simulink model "InjCrv_PoI2AddCor"  (R2016b)
settings: configuration reference "CodeGenConfigSet" (kept outside this file)
values from neighbouring files (symbols this model uses):
  ETCtl_qPoI2_C = Calibration.Parameter    [init_InjCrv_PoI2AddCor.m]
  InjCrv_phiAddCorRmt_C = Calibration.Parameter    [init_InjCrv_PoI2AddCor.m]
  InjCrv_phiPoI2_C = Calibration.Parameter    [init_InjCrv_PoI2AddCor.m]
  InjCrv_qPoI2_C = Calibration.Parameter    [init_InjCrv_PoI2AddCor.m]
  InjCrv_qPoI2Eff_C = Calibration.Parameter    [init_InjCrv_PoI2AddCor.m]
  InjCrv_stInjCharSetVal_C = Calibration.Parameter    [init_InjCrv_PoI2AddCor.m]
  InjCrv_swtPhiAddCorRmt_C = Calibration.Parameter    [init_InjCrv_PoI2AddCor.m]
  InjCrv_swtPoI2ETCtl_C = Calibration.Parameter    [init_InjCrv_PoI2AddCor.m]
  InjCrv_swtPoI2FMTC_C = Calibration.Parameter    [init_InjCrv_PoI2AddCor.m]
  InjCrv_swtPoI2Phi_C = Calibration.Parameter    [init_InjCrv_PoI2AddCor.m]
  InjCrv_swtPoI2Q_C = Calibration.Parameter    [init_InjCrv_PoI2AddCor.m]
  InjCrv_swtPoI2QEff_C = Calibration.Parameter    [init_InjCrv_PoI2AddCor.m]
  InjCrv_swtPoI2Ti_C = Calibration.Parameter    [init_InjCrv_PoI2AddCor.m]
  InjCrv_swtTiAddCorRmt_C = Calibration.Parameter    [init_InjCrv_PoI2AddCor.m]
  InjCrv_tiAddCorRmt_C = Calibration.Parameter    [init_InjCrv_PoI2AddCor.m]
  InjCrv_tiPoI2_C = Calibration.Parameter    [init_InjCrv_PoI2AddCor.m]
undefined symbols (not defined in the file or in its folder): Switch_conv
libraries: simulink x2
settings Model: Creator=Administrator  LastModifiedBy=Wei Liang
settings ConfigSetRef: SourceLocation=Base Workspace

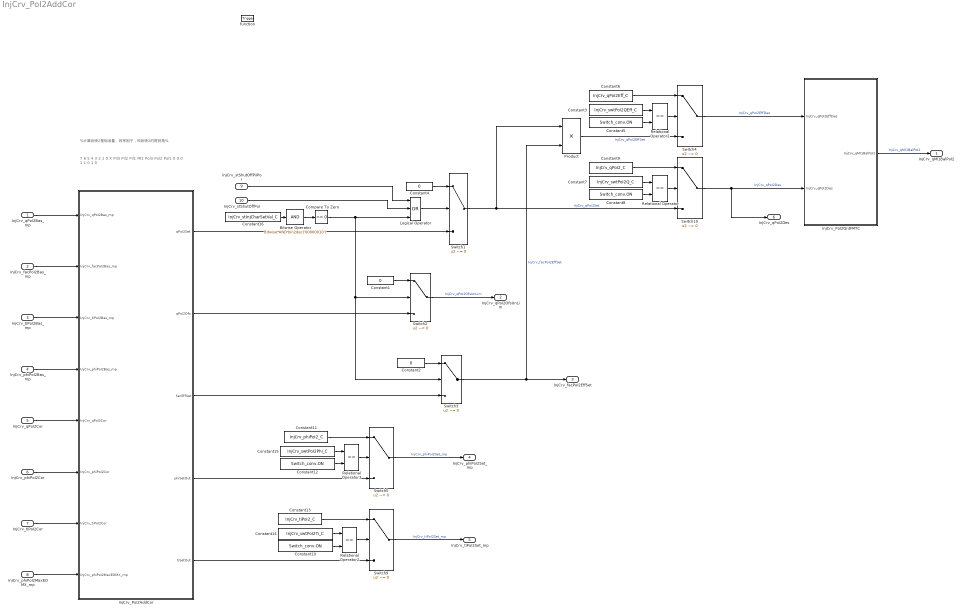
== system InjCrv_PoI2AddCor ==
  note: %计算后喷2基础油量，效率因子，和后喷2的提前角%
  note: 7
      | 6
      | 5
      | 4
      | 3
      | 2
      | 1
      | 0
      |
      | X
      | Pil3
      | Pil2
      | Pil1
      | MI1
      | Pol3
      | Pol2
      | Pol1
      |
      | 0
      | 0
      | 0
      | 1
      | 1
      | 0
      | 1
      | 0
  InjCrv_qPoI2Bas_mp : Inport  Tag=mg/hub  Description=PoI2 base quantity for injection  OutMin=-319  OutMax=319  OutDataTypeStr=FuelMass_mg_hub
  InjCrv_facPoI2Bas_mp : Inport  Description=PoI2 base Efficiency factor  Port=2  OutMin=-10  OutMax=10  OutDataTypeStr=Factor
  InjCrv_tiPoI2Bas_mp : Inport  Tag=us  Description=PoI2 base start of energizing of time  Port=3  OutMin=-13107  OutMax=13106  OutDataTypeStr=InjTime_us
  InjCrv_phiPoI2Bas_mp : Inport  Tag=CA  Description=PoI2 base start of energizing of angle  Port=4  OutMin=-719  OutMax=719  OutDataTypeStr=Angle_CA
  InjCrv_qPoI2Cor : Inport  Tag=mg/hub  Description=PoI2 correction quantity  Port=5  OutMin=-319  OutMax=319  OutDataTypeStr=FuelMass_mg_hub
  InjCrv_phiPoI2Cor : Inport  Tag=CA  Description=PoI2 start of energizing correction angle  Port=6  OutMin=-719  OutMax=719  OutDataTypeStr=Angle_CA
  InjCrv_tiPoI2Cor : Inport  Tag=us  Description=PoI2 start of energizing correction time  Port=7  OutMin=-13107  OutMax=13106  OutDataTypeStr=InjTime_us
  InjCrv_phiPoI2MaxEOMX_mp : Inport  Tag=CA  Description=Maximum PoI2 start of energizing for EOM1-EOM7  Port=8  OutMin=-719  OutMax=719  OutDataTypeStr=Angle_CA
  InjCrv_stShutOffPiIPoI : Inport  Description=State of MI1 fuelMass too small  Port=9  OutMin=0  OutMax=1  OutDataTypeStr=boolean
  InjCrv_stShutOffPoI : Inport  Description=State of MI1 fuelMass too small  Port=10  OutMin=0  OutMax=1  OutDataTypeStr=boolean
  function : TriggerPort  TriggerType=function-call  VariantControl=Variant
  Bitwise Operator : simulink/Logic and Bit Operations/Bitwise Operator  logicop=AND  UseBitMask=on  BitMask=bin2dec('00000010')  BitMaskRealWorld=Stored Integer
  Compare To Zero : simulink/Logic and Bit Operations/Compare To Zero  relop===  OutDataTypeStr=boolean
  Constant1 : Constant  Value=0  OutDataTypeStr=Inherit: Inherit via back propagation
  Constant{5,8,10,12} (4 alike) : Constant  Value=Switch_conv.ON
  Constant11 : Constant  Value=InjCrv_phiPoI2_C
  Constant13 : Constant  Value=InjCrv_tiPoI2_C
  Constant14 : Constant  Value=InjCrv_swtPoI2Ti_C
  Constant15 : Constant  Value=InjCrv_swtPoI2Phi_C
  Constant16 : Constant  Value=InjCrv_stInjCharSetVal_C
  Constant2 : Constant  Value=0  OutDataTypeStr=Inherit: Inherit via back propagation
  Constant3 : Constant  Value=InjCrv_swtPoI2QEff_C
  Constant4 : Constant  Value=0  OutDataTypeStr=Inherit: Inherit via back propagation
  Constant6 : Constant  Value=InjCrv_qPoI2Eff_C
  Constant7 : Constant  Value=InjCrv_swtPoI2Q_C
  Constant9 : Constant  Value=InjCrv_qPoI2_C
  InjCrv_PoI2AddCor : Subsystem  RTWFcnName=InjCrv_PoI2AddCor_Co  RTWFileName=InjCrv_PoI2AddCor
      settings: RTWSystemCode=Nonreusable function  RTWFcnNameOpts=User specified  RTWFileNameOpts=User specified
  InjCrv_PoI2QntFMTC : Subsystem
  Logical Operator : Logic  Operator=OR  Inputs=3  AllPortsSameDT=off  OutDataTypeStr=boolean
  Product : Product  OutDataTypeStr=Inherit: Inherit via back propagation  SaturateOnIntegerOverflow=on
  Relational Operator{,1..3} (4 alike) : RelationalOperator  Operator===  OutDataTypeStr=boolean  RndMeth=Simplest
  Switch{1..5,9..10} (7 alike) : Switch  Criteria=u2 ~= 0
  InjCrv_qMI1BalPoI2 : Outport  Tag=mg/hub  Description=Actual PoI2 quantity contained in FMTC (used for MI1 balance)  OutMin=-319  OutMax=319  OutDataTypeStr=FuelMass_mg_hub
  InjCrv_qPoI2OfsUnLim : Outport  Tag=mg/hub  Description=Unlimited PoI2 offset quantity  Port=2  OutMin=-319  OutMax=319  OutDataTypeStr=FuelMass_mg_hub
  InjCrv_facPoI2EffSet : Outport  Description=Factor for torque forming part of PoI2 injection quantity (setpoint)  Port=3  OutMin=-10  OutMax=10  OutDataTypeStr=Factor
  InjCrv_phiPoI2Set_mp : Outport  Tag=CA  Description=start of energizing Agngle for PoI2  Port=4  OutMin=-719  OutMax=719  OutDataTypeStr=Angle_CA
  InjCrv_tiPoI2Set_mp : Outport  Tag=us  Description=start of energizing time for PoI2  Port=5  OutMin=-13107  OutMax=13106  OutDataTypeStr=InjTime_us
  InjCrv_qPoI2Des : Outport  Tag=mg/hub  Description=Desired PoI2 injection quantity  Port=6  OutMin=-319  OutMax=319  OutDataTypeStr=FuelMass_mg_hub
  wires:
  InjCrv_qPoI2Cor/1 -> InjCrv_PoI2AddCor/5(InjCrv_qPoI2Cor)
  InjCrv_phiPoI2Cor/1 -> InjCrv_PoI2AddCor/6(InjCrv_phiPoI2Cor)
  InjCrv_tiPoI2Cor/1 -> InjCrv_PoI2AddCor/7(InjCrv_tiPoI2Cor)
  InjCrv_PoI2AddCor/1(qPoI2Set) -> Switch1/3
  Switch5/1 -> InjCrv_phiPoI2Set_mp/1  "InjCrv_phiPoI2Set_mp"
  Switch9/1 -> InjCrv_tiPoI2Set_mp/1  "InjCrv_tiPoI2Set_mp"
  Switch1/1 -> Product/1, Switch10/3  "InjCrv_qPoI2Set"
  Bitwise Operator/1 -> Compare To Zero/1
  Constant16/1 -> Bitwise Operator/1
  Constant4/1 -> Switch1/1
  Switch2/1 -> InjCrv_qPoI2OfsUnLim/1  "InjCrv_qPoI2OfsUnLim"
  InjCrv_PoI2AddCor/2(qPoI2Ofs) -> Switch2/3
  InjCrv_PoI2AddCor/3(facEffSet) -> Switch3/3
  Switch3/1 -> InjCrv_facPoI2EffSet/1, Product/2  "InjCrv_facPoI2EffSet"
  Product/1 -> Switch4/3  "InjCrv_qPoI2EffSet"
  Constant6/1 -> Switch4/1
  Constant3/1 -> Relational Operator1/1
  Constant5/1 -> Relational Operator1/2
  Relational Operator1/1 -> Switch4/2
  Switch4/1 -> InjCrv_PoI2QntFMTC/1(InjCrv_qPoI2EffDes)  "InjCrv_qPoI2EffDes"
  Constant9/1 -> Switch10/1
  Constant7/1 -> Relational Operator/1
  Constant8/1 -> Relational Operator/2
  Relational Operator/1 -> Switch10/2
  Switch10/1 -> InjCrv_qPoI2Des/1, InjCrv_PoI2QntFMTC/2(InjCrv_qPoI2Des)  "InjCrv_qPoI2Des"
  Constant10/1 -> Relational Operator2/2
  Relational Operator2/1 -> Switch9/2
  Constant12/1 -> Relational Operator3/2
  Relational Operator3/1 -> Switch5/2
  InjCrv_PoI2AddCor/4(phiSetOut) -> Switch5/3
  InjCrv_PoI2AddCor/5(tiSetOut) -> Switch9/3
  Constant14/1 -> Relational Operator2/1
  Constant13/1 -> Switch9/1
  Constant11/1 -> Switch5/1
  Constant15/1 -> Relational Operator3/1
  Logical Operator/1 -> Switch1/2
  Compare To Zero/1 -> Logical Operator/3, Switch3/2, Switch2/2
  Constant1/1 -> Switch2/1
  Constant2/1 -> Switch3/1
  InjCrv_stShutOffPoI/1 -> Logical Operator/2
  InjCrv_stShutOffPiIPoI/1 -> Logical Operator/1
  InjCrv_PoI2QntFMTC/1(InjCrv_qMI1BalPoI2) -> InjCrv_qMI1BalPoI2/1  "InjCrv_qMI1BalPoI2"
  InjCrv_phiPoI2Bas_mp/1 -> InjCrv_PoI2AddCor/4(InjCrv_phiPoI2Bas_mp)
  InjCrv_tiPoI2Bas_mp/1 -> InjCrv_PoI2AddCor/3(InjCrv_tiPoI2Bas_mp)
  InjCrv_facPoI2Bas_mp/1 -> InjCrv_PoI2AddCor/2(InjCrv_facPoI2Bas_mp)
  InjCrv_qPoI2Bas_mp/1 -> InjCrv_PoI2AddCor/1(InjCrv_qPoI2Bas_mp)
  InjCrv_phiPoI2MaxEOMX_mp/1 -> InjCrv_PoI2AddCor/8(InjCrv_phiPoI2MaxEOMX_mp)

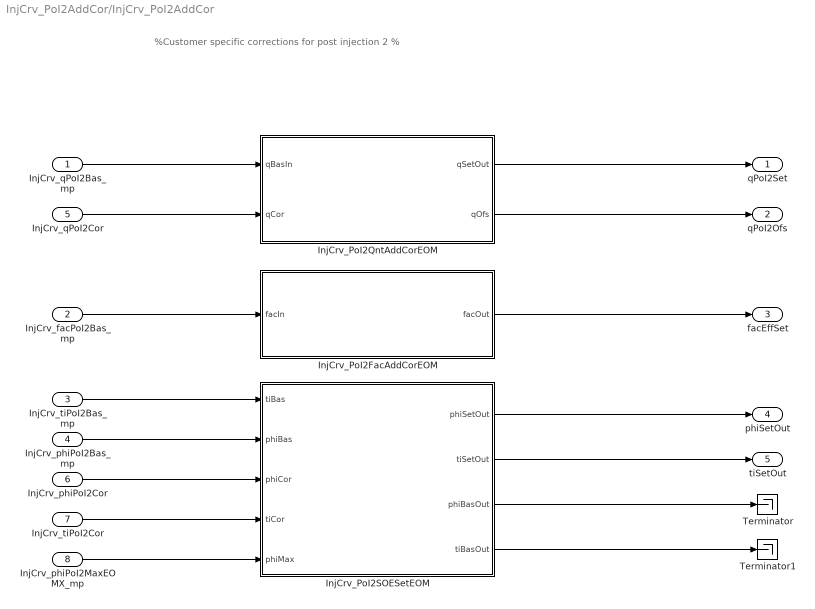
== system InjCrv_PoI2AddCor/InjCrv_PoI2AddCor ==
  note: %Customer specific corrections for post injection 2 %
  InjCrv_qPoI2Bas_mp : Inport
  InjCrv_facPoI2Bas_mp : Inport  Port=2
  InjCrv_tiPoI2Bas_mp : Inport  Port=3
  InjCrv_phiPoI2Bas_mp : Inport  Port=4
  InjCrv_qPoI2Cor : Inport  Port=5
  InjCrv_phiPoI2Cor : Inport  Port=6
  InjCrv_tiPoI2Cor : Inport  Port=7
  InjCrv_phiPoI2MaxEOMX_mp : Inport  Port=8
  InjCrv_PoI2FacAddCorEOM : Subsystem
  InjCrv_PoI2QntAddCorEOM : Subsystem
  InjCrv_PoI2SOESetEOM : Subsystem
  Terminator : Terminator
  Terminator1 : Terminator
  qPoI2Set : Outport
  qPoI2Ofs : Outport  Port=2
  facEffSet : Outport  Port=3
  phiSetOut : Outport  Port=4
  tiSetOut : Outport  Port=5
  wires:
  InjCrv_PoI2QntAddCorEOM/1(qSetOut) -> qPoI2Set/1
  InjCrv_qPoI2Bas_mp/1 -> InjCrv_PoI2QntAddCorEOM/1(qBasIn)
  InjCrv_qPoI2Cor/1 -> InjCrv_PoI2QntAddCorEOM/2(qCor)
  InjCrv_PoI2QntAddCorEOM/2(qOfs) -> qPoI2Ofs/1
  InjCrv_PoI2FacAddCorEOM/1(facOut) -> facEffSet/1
  InjCrv_facPoI2Bas_mp/1 -> InjCrv_PoI2FacAddCorEOM/1(facIn)
  InjCrv_PoI2SOESetEOM/1(phiSetOut) -> phiSetOut/1
  InjCrv_tiPoI2Bas_mp/1 -> InjCrv_PoI2SOESetEOM/1(tiBas)
  InjCrv_PoI2SOESetEOM/2(tiSetOut) -> tiSetOut/1
  InjCrv_phiPoI2Cor/1 -> InjCrv_PoI2SOESetEOM/3(phiCor)
  InjCrv_tiPoI2Cor/1 -> InjCrv_PoI2SOESetEOM/4(tiCor)
  InjCrv_PoI2SOESetEOM/3(phiBasOut) -> Terminator/1
  InjCrv_phiPoI2Bas_mp/1 -> InjCrv_PoI2SOESetEOM/2(phiBas)
  InjCrv_phiPoI2MaxEOMX_mp/1 -> InjCrv_PoI2SOESetEOM/5(phiMax)
  InjCrv_PoI2SOESetEOM/4(tiBasOut) -> Terminator1/1

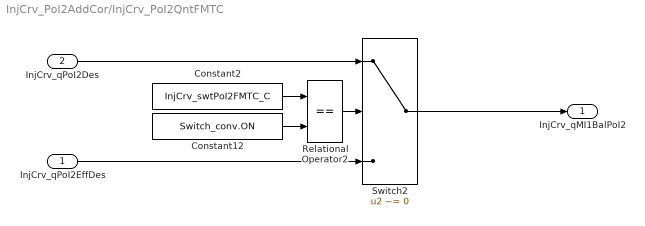
== system InjCrv_PoI2AddCor/InjCrv_PoI2QntFMTC ==
  InjCrv_qPoI2EffDes : Inport
  InjCrv_qPoI2Des : Inport  Port=2
  Constant12 : Constant  Value=Switch_conv.ON
  Constant2 : Constant  Value=InjCrv_swtPoI2FMTC_C
  Relational Operator2 : RelationalOperator  Operator===  OutDataTypeStr=boolean  RndMeth=Simplest
  Switch2 : Switch  Criteria=u2 ~= 0
  InjCrv_qMI1BalPoI2 : Outport
  wires:
  InjCrv_qPoI2EffDes/1 -> Switch2/3
  Constant2/1 -> Relational Operator2/1
  InjCrv_qPoI2Des/1 -> Switch2/1
  Switch2/1 -> InjCrv_qMI1BalPoI2/1
  Constant12/1 -> Relational Operator2/2
  Relational Operator2/1 -> Switch2/2

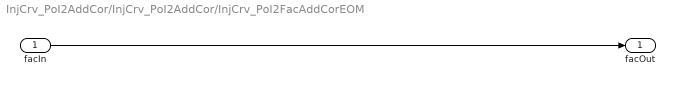
== system InjCrv_PoI2AddCor/InjCrv_PoI2AddCor/InjCrv_PoI2FacAddCorEOM ==
  facIn : Inport
  facOut : Outport
  wires:
  facIn/1 -> facOut/1

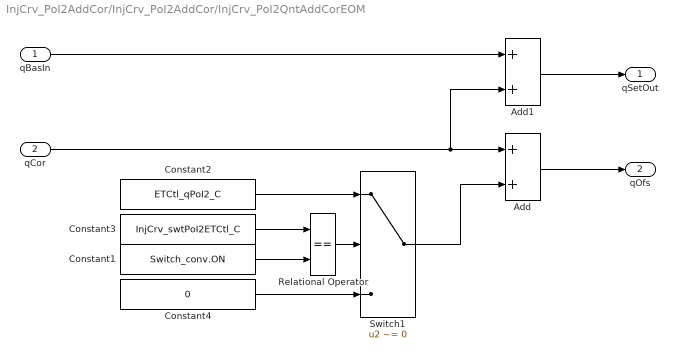
== system InjCrv_PoI2AddCor/InjCrv_PoI2AddCor/InjCrv_PoI2QntAddCorEOM ==
  qBasIn : Inport
  qCor : Inport  Port=2
  Add : Sum  SaturateOnIntegerOverflow=on
  Add1 : Sum  SaturateOnIntegerOverflow=on
  Constant1 : Constant  Value=Switch_conv.ON
  Constant2 : Constant  Value=ETCtl_qPoI2_C
  Constant3 : Constant  Value=InjCrv_swtPoI2ETCtl_C
  Constant4 : Constant  Value=0  OutDataTypeStr=Inherit: Inherit via back propagation
  Relational Operator : RelationalOperator  Operator===  OutDataTypeStr=boolean  RndMeth=Simplest
  Switch1 : Switch  Criteria=u2 ~= 0
  qSetOut : Outport
  qOfs : Outport  Port=2
  wires:
  qCor/1 -> Add1/2, Add/1
  qBasIn/1 -> Add1/1
  Relational Operator/1 -> Switch1/2
  Constant3/1 -> Relational Operator/1
  Constant1/1 -> Relational Operator/2
  Constant2/1 -> Switch1/1
  Constant4/1 -> Switch1/3
  Switch1/1 -> Add/2
  Add/1 -> qOfs/1
  Add1/1 -> qSetOut/1

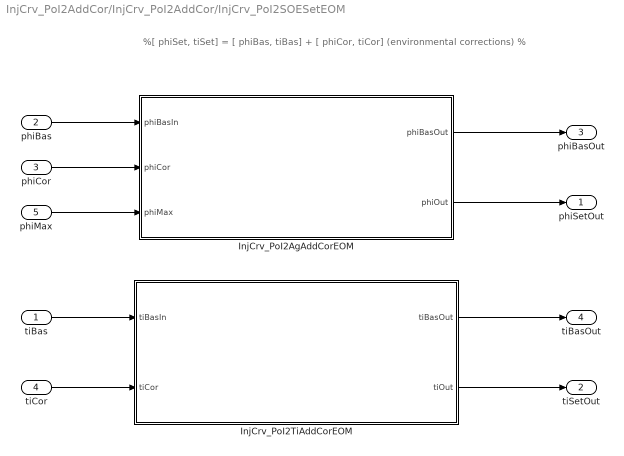
== system InjCrv_PoI2AddCor/InjCrv_PoI2AddCor/InjCrv_PoI2SOESetEOM ==
  note: %[ phiSet, tiSet] = [ phiBas, tiBas] + [ phiCor, tiCor] (environmental corrections) %
  tiBas : Inport
  phiBas : Inport  Port=2
  phiCor : Inport  Port=3
  tiCor : Inport  Port=4
  phiMax : Inport  Port=5
  InjCrv_PoI2AgAddCorEOM : Subsystem
  InjCrv_PoI2TiAddCorEOM : Subsystem
  phiSetOut : Outport
  tiSetOut : Outport  Port=2
  phiBasOut : Outport  Port=3
  tiBasOut : Outport  Port=4
  wires:
  phiBas/1 -> InjCrv_PoI2AgAddCorEOM/1(phiBasIn)
  phiCor/1 -> InjCrv_PoI2AgAddCorEOM/2(phiCor)
  tiBas/1 -> InjCrv_PoI2TiAddCorEOM/1(tiBasIn)
  tiCor/1 -> InjCrv_PoI2TiAddCorEOM/2(tiCor)
  InjCrv_PoI2AgAddCorEOM/1(phiBasOut) -> phiBasOut/1
  InjCrv_PoI2TiAddCorEOM/1(tiBasOut) -> tiBasOut/1
  InjCrv_PoI2AgAddCorEOM/2(phiOut) -> phiSetOut/1
  InjCrv_PoI2TiAddCorEOM/2(tiOut) -> tiSetOut/1
  phiMax/1 -> InjCrv_PoI2AgAddCorEOM/3(phiMax)

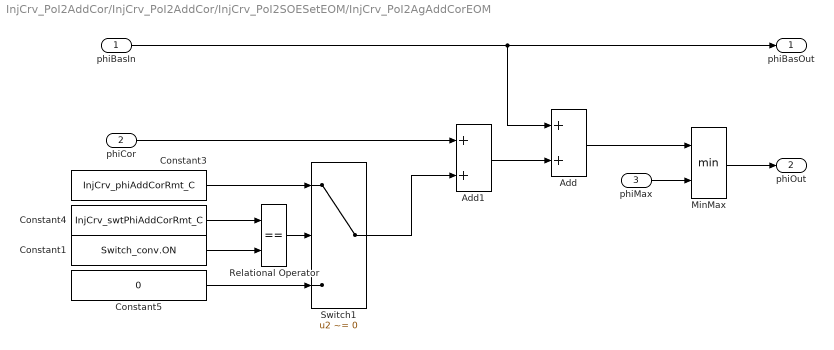
== system InjCrv_PoI2AddCor/InjCrv_PoI2AddCor/InjCrv_PoI2SOESetEOM/InjCrv_PoI2AgAddCorEOM ==
  phiBasIn : Inport
  phiCor : Inport  Port=2
  phiMax : Inport  Port=3
  Add : Sum  SaturateOnIntegerOverflow=on  InputSameDT=on
  Add1 : Sum  SaturateOnIntegerOverflow=on  InputSameDT=on
  Constant1 : Constant  Value=Switch_conv.ON
  Constant3 : Constant  Value=InjCrv_phiAddCorRmt_C
  Constant4 : Constant  Value=InjCrv_swtPhiAddCorRmt_C
  Constant5 : Constant  Value=0  OutDataTypeStr=Inherit: Inherit via back propagation
  MinMax : MinMax  Inputs=2  InputSameDT=on
  Relational Operator : RelationalOperator  Operator===  OutDataTypeStr=boolean  RndMeth=Simplest
  Switch1 : Switch  Criteria=u2 ~= 0
  phiBasOut : Outport
  phiOut : Outport  Port=2
  wires:
  phiCor/1 -> Add1/1
  phiBasIn/1 -> Add/1, phiBasOut/1
  Relational Operator/1 -> Switch1/2
  Constant4/1 -> Relational Operator/1
  Constant1/1 -> Relational Operator/2
  Constant3/1 -> Switch1/1
  Constant5/1 -> Switch1/3
  Switch1/1 -> Add1/2
  Add1/1 -> Add/2
  Add/1 -> MinMax/1
  phiMax/1 -> MinMax/2
  MinMax/1 -> phiOut/1

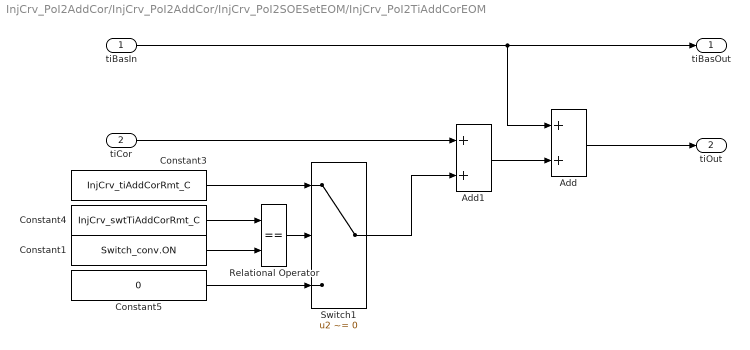
== system InjCrv_PoI2AddCor/InjCrv_PoI2AddCor/InjCrv_PoI2SOESetEOM/InjCrv_PoI2TiAddCorEOM ==
  tiBasIn : Inport
  tiCor : Inport  Port=2
  Add : Sum  SaturateOnIntegerOverflow=on  InputSameDT=on
  Add1 : Sum  SaturateOnIntegerOverflow=on  InputSameDT=on
  Constant1 : Constant  Value=Switch_conv.ON
  Constant3 : Constant  Value=InjCrv_tiAddCorRmt_C
  Constant4 : Constant  Value=InjCrv_swtTiAddCorRmt_C
  Constant5 : Constant  Value=0  OutDataTypeStr=Inherit: Inherit via back propagation
  Relational Operator : RelationalOperator  Operator===  OutDataTypeStr=boolean  RndMeth=Simplest
  Switch1 : Switch  Criteria=u2 ~= 0
  tiBasOut : Outport
  tiOut : Outport  Port=2
  wires:
  tiCor/1 -> Add1/1
  tiBasIn/1 -> tiBasOut/1, Add/1
  Relational Operator/1 -> Switch1/2
  Constant4/1 -> Relational Operator/1
  Constant1/1 -> Relational Operator/2
  Constant3/1 -> Switch1/1
  Constant5/1 -> Switch1/3
  Switch1/1 -> Add1/2
  Add1/1 -> Add/2
  Add/1 -> tiOut/1
